simulink model "lab4"  (R2017b)
settings: Solver=ode4  StartTime=0.0  StopTime=10.0  FixedStep=0.0001  RelTol=1e-3
undefined symbols (not defined in the file or in its folder): C, R
settings Model: Creator=ayushi  LastModifiedBy=ayushi

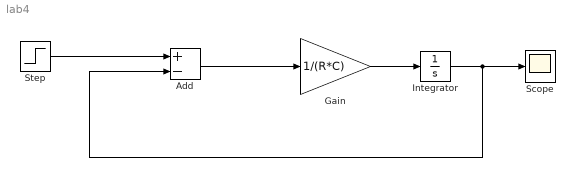
== system lab4 ==
  Add : Sum  Inputs=+-
  Gain : Gain  Gain=1/(R*C)
  Integrator : Integrator
  Scope : Scope
  Step : Step  SampleTime=0
  wires:
  Step/1 -> Add/1
  Add/1 -> Gain/1
  Integrator/1 -> Add/2, Scope/1
  Gain/1 -> Integrator/1
